simulink model "untitled"  (R2013b)
settings: Solver=ode45  StartTime=0.0  StopTime=10.0  RelTol=1e-3
values from neighbouring files (symbols this model uses):
  A = [0 0 0; 1 0 -1; 0 1 2]    [SLN.m]    (also in exe1.m = [0, 0, 0; 1, 0, -1; 0, 1, 2])
  B = [0 -1; 1 0; 0 1]    [SLN.m]    (also in exe1.m = [0 -1;1 0;0 1])
  C = [1 0 1]    [SLN.m]    (also in exe1.m)
  F = F0+g0*f_t    [SLN.m]    (also in exe1.m = F0 + g*f_t)
  G = eye(p)    [SLN.m]    (also in exe1.m = eye(2))
settings Model: Creator=Student  LastModifiedBy=Student

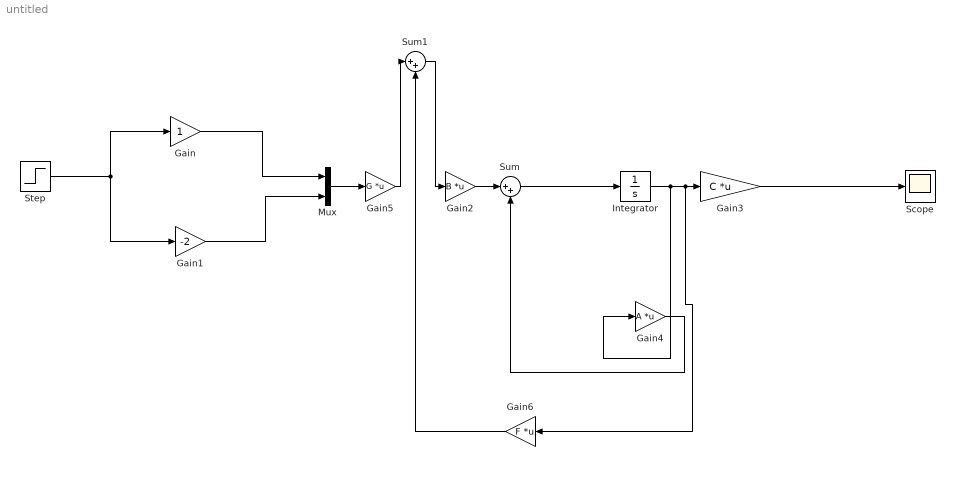
== system untitled ==
  Gain : Gain
  Gain1 : Gain  Gain=-2  SampleTime=1
  Gain2 : Gain  Gain=B  Multiplication=Matrix(K*u)
  Gain3 : Gain  Gain=C  Multiplication=Matrix(K*u)
  Gain4 : Gain  Gain=A  Multiplication=Matrix(K*u)
  Gain5 : Gain  Gain=G  Multiplication=Matrix(K*u)
  Gain6 : Gain  Gain=F  Multiplication=Matrix(K*u)
  Integrator : Integrator
  Mux : Mux  Inputs=2
  Scope : Scope
  Step : Step  SampleTime=0
  Sum : Sum  Inputs=|++
  Sum1 : Sum  Inputs=|++
  wires:
  Step/1 -> Gain/1, Gain1/1
  Gain/1 -> Mux/1
  Gain1/1 -> Mux/2
  Gain2/1 -> Sum/1
  Sum/1 -> Integrator/1
  Integrator/1 -> Gain4/1, Gain6/1, Gain3/1
  Gain4/1 -> Sum/2
  Gain3/1 -> Scope/1
  Mux/1 -> Gain5/1
  Gain5/1 -> Sum1/1
  Sum1/1 -> Gain2/1
  Gain6/1 -> Sum1/2
